simulink library "EdgePorts"  (R2022b)
settings: Solver=VariableStepAuto  StartTime=0.0  StopTime=10.0  RelTol=1e-3
libraries: HandyTextFile x5, AudioStats x4, $bdroot x2, TalariaApiBuffer x2
settings Model: Creator=kl13806  LastModifiedBy=kl13806
settings SolverCC: AlgebraicLoopSolver=TrustRegion
settings DebuggingCC: UnconnectedInputMsg=warning  UnconnectedOutputMsg=warning  UnconnectedLineMsg=warning  SFMachineParentedDataDiag=warning
settings ModelReferenceCC: EnableRefExpFcnMdlSchedulingChecks=on
settings RTWCC: DLArmComputeVersion=19.05

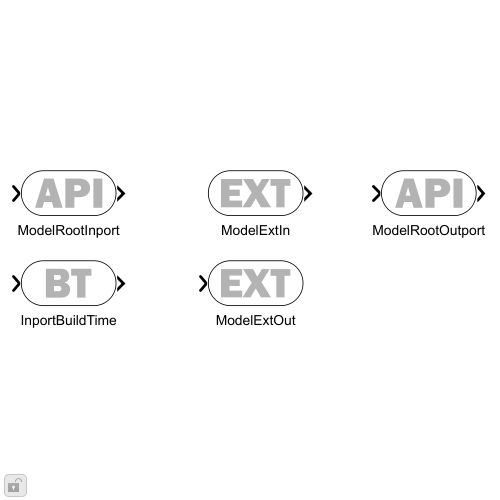
[thumbnail: Simulink's stored preview of the top-level diagram]
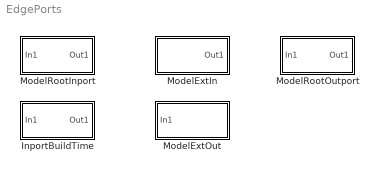
== system EdgePorts ==
  InportBuildTime : Subsystem  mask(Talaria Build-Time Configured Inport){Config=[]}
      mask prompts: Config "InportBuildTimeConfig"
      mask help: This block is just an inport with its signal attributes controlled by a build-time configuration object of type InportBTConfig.
      mask init:
      | blkh=gcbh;
      | Config=BTConfig.Assert(blkh,Config);
      | 
      | Config.Validate();
      mask Help: Supply the name of variable of type InportBTConfig in the mask dialog. Supplying empty (i.e. [ ]) will use class defaults which may change over time.
      mask Display: image('InportBT_Mask.svg'); % Use "Edit Image" on toolstrip to change.
  ModelExtIn : Subsystem  mask(Talaria Model External Inport){Config=[]}
      mask prompts: Config "ModelExtInConfig"
      mask help: This block acts like an inport and generates DLL API code.
      mask init:
      | blkh=gcbh;
      | Config=BTConfig.Assert(blkh,Config);
      | 
      | Config.Validate();
      mask Help:
      | The Talaria Model External Inport block assists with running algorithms which are built into DLLs. This block acts like an inport and exposes an API designed to feed data into the model. A driving program (e.g. a tuning tool) can use this standard interface to run any algorithm that uses this block.
      | 
      | See ext_port_model.m for an example of how to interface with the generated DLL. Also check the generated TalariaAPI.h source file.
      mask Display: image('ModelExtMask.svg'); % Use "Edit Image" on toolstrip to change.
  ModelExtOut : Subsystem  mask(Talaria Model External Outport){BufferName='Out1'}
      mask prompts: BufferName "Buffer Name:"
      mask help: This block acts like an outport and generates DLL API code.
      mask Help:
      | The Talaria Model External Outport block assists with running algorithms which are built into DLLs. This block acts like an outport and exposes an API designed to retrieve the data emit from the model. A driving program (e.g. a tuning tool) can use this standard interface to run any algorithm that uses this block.
      | 
      | See ext_port_model.m for an example of how to interface with the generated DLL. Also check the generated TalariaAPI.h source file.
      mask Display: image('ModelExtMask.svg'); % Use "Edit Image" on toolstrip to change.
  ModelRootInport : Subsystem  mask(Talaria Model Root Inport){Config=[]}
      mask prompts: Config "ModelRootInportConfig"
      mask help: This block controls the signal attributes, name, and storage class of attached buffer in the generated code. Also the buffer is surfaced as a model-level integration point (e.g. TalariaAPI.h, etc)
      mask init:
      | blkh=gcbh;
      | Config=BTConfig.Assert(blkh,Config);
      | 
      | Config.Validate();
      mask Help:
      | This block is intended to be used for root-block-diagram ports in an application model. Driven by built-time configuration, it sets up the input buffer's signal attributes, the type of buffer (e.g. extern pointer vs. exported model-allocated), and adds these specfications to the generated code in TalariaAPI.h.
      | 
      | Make sure to feed this block with just a normal Simulink root-level inport with no signal attributes settings made to it. All the configuration settings are asserted inside this block.
      mask Display: image('ModelRootInportMask.svg'); % Use "Edit Image" on toolstrip to change.
  ModelRootOutport : Subsystem  mask(Talaria Model Root Outport){Config=[]}
      mask prompts: Config "ModelRootOutportConfig"
      mask help: This block controls the name and storage class of attached buffer in the generated code. Also the buffer is surfaced as a model-level integration point (e.g. TalariaAPI.h, etc)
      mask init:
      | blkh=gcbh;
      | Config=BTConfig.Assert(blkh,Config);
      | 
      | Config.Validate();
      mask Help:
      | This block is intended to be used for root-block-diagram ports in an application model. Driven by built-time configuration, it sets up the output buffer qualities such as the type of buffer (e.g. extern pointer vs. exported model-allocated), and adds the discovered signal specfications to the generated code in TalariaAPI.h.
      | 
      | Note that this block does *not* control the signal attributes of the buffer such as data type, dimensions, and sample time.
      mask Display: image('ModelRootInportMask.svg'); % Use "Edit Image" on toolstrip to change.

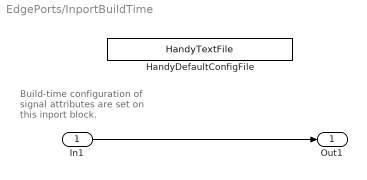
== system EdgePorts/InportBuildTime ==
  note: Build-time configuration of
      | signal attributes are set on
      | this inport block.
  In1 : Inport  OutDataTypeStr=Config.DataType  PortDimensions=Config.Dimensions  SampleTime=Config.SampleTime
  HandyDefaultConfigFile : HandyTextFile/HandyTextFile  TemplateSource=Config  FileSuffix=Config.m  OpenDialogOnLoad=off  UseThisBlockName=off  TheDefaultText=|  ShowInLibBrowser=on
      | classdef $(PREFIX)$(SUFFIX)
      | % $(FILENAME) Class definition to contain build-time configuration for $(PREFIX)
      | % Usage:
      | %    aConfig = $(PREFIX)$(SUFFIX)
      | %
      | 
      | %   Copyright 2020 Bose Corporation
      | 
      |   properties
      |     % Properties use this syntax:
      |     %    PropertyName size class {validation functions} = DefaultValue
      |     % About Build-Time Configuration: https://wiki.bose.com/x/dqPoB
      | 
      |     % Delete these examples:
      |     %Gain = 0.5
      |     %Theta = sin(pi/12)
      |     %MyDoubleArray (1,7) double {mustBeFinite} = [1 2 3 4 5 6 7]
      |     %LeftConfig (1,1) SubBlockConfig
      |     %RightConfig (1,1) SubBlockConfig
      | 
      |   end
      | end
      settings: SourceProductName=Bose Talaria
  Out1 : Outport
  wires:
  In1/1 -> Out1/1

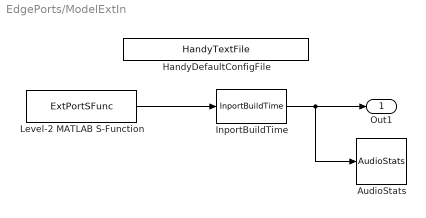
== system EdgePorts/ModelExtIn ==
  AudioStats : AudioStats/AudioStats  DoSampleRate=off  TypeSampleRate=Inherit: auto  DoCallRate=off  TypeCallRate=Inherit: auto  DoFrameSize=off  TypeFrameSize=Inherit: auto  DoChannelCount=off  TypeChannelCount=Inherit: auto  DoTaskRateFactor=off  TypeTaskRateFactor=Inherit: auto  MacroNameRoot=AUDIO  MacroNameRootEval=Config.BufferName  IsMacroNameEval=on  MacroSampleRate=on  MacroCallRate=on  MacroFrameSize=on  MacroChannelCount=on  MacroTaskRateFactor=on  MacroTaskId=on  ValidateSampleRate=off  ValueSampleRate=[]  ValidateCallRate=off  ValueCallRate=[]  ValidateFrameSize=off  ValueFrameSize=[]  ValidateChannelCount=off  ValueChannelCount=[]  ValidateTaskRateFactor=off  ValueTaskRateFactor=[]
      settings: SourceProductName=Bose Talaria
  HandyDefaultConfigFile : HandyTextFile/HandyTextFile  TemplateSource=Config  FileSuffix=Config.m  OpenDialogOnLoad=off  UseThisBlockName=off  TheDefaultText=|  ShowInLibBrowser=on
      | classdef $(PREFIX)$(SUFFIX)
      | % $(FILENAME) Class definition to contain build-time configuration for $(PREFIX)
      | % Usage:
      | %    aConfig = $(PREFIX)$(SUFFIX)
      | %
      | 
      | %   Copyright 2020 Bose Corporation
      | 
      |   properties
      |     % Properties use this syntax:
      |     %    PropertyName size class {validation functions} = DefaultValue
      |     % About Build-Time Configuration: https://wiki.bose.com/x/dqPoB
      | 
      |     % Delete these examples:
      |     %Gain = 0.5
      |     %Theta = sin(pi/12)
      |     %MyDoubleArray (1,7) double {mustBeFinite} = [1 2 3 4 5 6 7]
      |     %LeftConfig (1,1) SubBlockConfig
      |     %RightConfig (1,1) SubBlockConfig
      | 
      |   end
      | end
      settings: SourceProductName=Bose Talaria
  InportBuildTime : $bdroot/InportBuildTime  Config=Config
  Level-2 MATLAB S-Function : M-S-Function  FunctionName=ExtPortSFunc  Parameters=Config.BufferName,1
  Out1 : Outport
  wires:
  Level-2 MATLAB S-Function/1 -> InportBuildTime/1
  InportBuildTime/1 -> AudioStats/1, Out1/1

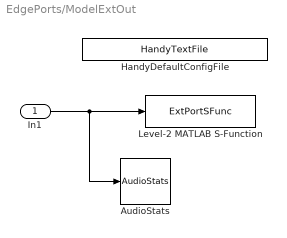
== system EdgePorts/ModelExtOut ==
  In1 : Inport
  AudioStats : AudioStats/AudioStats  DoSampleRate=off  TypeSampleRate=Inherit: auto  DoCallRate=off  TypeCallRate=Inherit: auto  DoFrameSize=off  TypeFrameSize=Inherit: auto  DoChannelCount=off  TypeChannelCount=Inherit: auto  DoTaskRateFactor=off  TypeTaskRateFactor=Inherit: auto  MacroNameRoot=AUDIO  MacroNameRootEval=BufferName  IsMacroNameEval=on  MacroSampleRate=on  MacroCallRate=on  MacroFrameSize=on  MacroChannelCount=on  MacroTaskRateFactor=on  MacroTaskId=on  ValidateSampleRate=off  ValueSampleRate=[]  ValidateCallRate=off  ValueCallRate=[]  ValidateFrameSize=off  ValueFrameSize=[]  ValidateChannelCount=off  ValueChannelCount=[]  ValidateTaskRateFactor=off  ValueTaskRateFactor=[]
      settings: SourceProductName=Bose Talaria
  HandyDefaultConfigFile : HandyTextFile/HandyTextFile  TemplateSource=Config  FileSuffix=Config.m  OpenDialogOnLoad=off  UseThisBlockName=off  TheDefaultText=|  ShowInLibBrowser=on
      | classdef $(PREFIX)$(SUFFIX)
      | % $(FILENAME) Class definition to contain build-time configuration for $(PREFIX)
      | % Usage:
      | %    aConfig = $(PREFIX)$(SUFFIX)
      | %
      | 
      | %   Copyright 2020 Bose Corporation
      | 
      |   properties
      |     % Properties use this syntax:
      |     %    PropertyName size class {validation functions} = DefaultValue
      |     % About Build-Time Configuration: https://wiki.bose.com/x/dqPoB
      | 
      |     % Delete these examples:
      |     %Gain = 0.5
      |     %Theta = sin(pi/12)
      |     %MyDoubleArray (1,7) double {mustBeFinite} = [1 2 3 4 5 6 7]
      |     %LeftConfig (1,1) SubBlockConfig
      |     %RightConfig (1,1) SubBlockConfig
      | 
      |   end
      | end
      settings: SourceProductName=Bose Talaria
  Level-2 MATLAB S-Function : M-S-Function  FunctionName=ExtPortSFunc  Parameters=BufferName,0
  wires:
  In1/1 -> AudioStats/1, Level-2 MATLAB S-Function/1

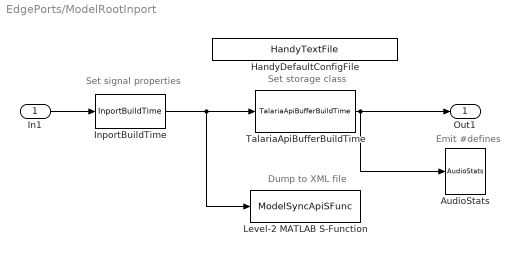
== system EdgePorts/ModelRootInport ==
  note: Dump to XML file
  note: Set storage class
  note: Set signal properties
  note: Emit #defines
  In1 : Inport
  AudioStats : AudioStats/AudioStats  DoSampleRate=off  TypeSampleRate=Inherit: auto  DoCallRate=off  TypeCallRate=Inherit: auto  DoFrameSize=off  TypeFrameSize=Inherit: auto  DoChannelCount=off  TypeChannelCount=Inherit: auto  DoTaskRateFactor=off  TypeTaskRateFactor=Inherit: auto  MacroNameRoot=AUDIO  MacroNameRootEval=Config.BufferName  IsMacroNameEval=on  MacroSampleRate=on  MacroCallRate=on  MacroFrameSize=on  MacroChannelCount=on  MacroTaskRateFactor=on  MacroTaskId=on  ValidateSampleRate=off  ValueSampleRate=[]  ValidateCallRate=off  ValueCallRate=[]  ValidateFrameSize=off  ValueFrameSize=[]  ValidateChannelCount=off  ValueChannelCount=[]  ValidateTaskRateFactor=off  ValueTaskRateFactor=[]
      settings: SourceProductName=Bose Talaria
  HandyDefaultConfigFile : HandyTextFile/HandyTextFile  TemplateSource=Config  FileSuffix=Config.m  OpenDialogOnLoad=off  UseThisBlockName=off  TheDefaultText=|  ShowInLibBrowser=on
      | classdef $(PREFIX)$(SUFFIX)
      | % $(FILENAME) Class definition to contain build-time configuration for $(PREFIX)
      | % Usage:
      | %    aConfig = $(PREFIX)$(SUFFIX)
      | %
      | 
      | %   Copyright 2020 Bose Corporation
      | 
      |   properties
      |     % Properties use this syntax:
      |     %    PropertyName size class {validation functions} = DefaultValue
      |     % About Build-Time Configuration: https://wiki.bose.com/x/dqPoB
      | 
      |     % Delete these examples:
      |     %Gain = 0.5
      |     %Theta = sin(pi/12)
      |     %MyDoubleArray (1,7) double {mustBeFinite} = [1 2 3 4 5 6 7]
      |     %LeftConfig (1,1) SubBlockConfig
      |     %RightConfig (1,1) SubBlockConfig
      | 
      |   end
      | end
      settings: SourceProductName=Bose Talaria
  InportBuildTime : $bdroot/InportBuildTime  Config=Config
  Level-2 MATLAB S-Function : M-S-Function  FunctionName=ModelSyncApiSFunc  Parameters=Config.BufferName,1,char(Config.AccessType)
  TalariaApiBufferBuildTime : TalariaApiBuffer/TalariaApiBufferBuildTime  Config=Config  TriggerInit=[415 69 515 111]
      settings: SourceProductName=Bose Talaria
  Out1 : Outport
  wires:
  In1/1 -> InportBuildTime/1
  InportBuildTime/1 -> Level-2 MATLAB S-Function/1, TalariaApiBufferBuildTime/1
  TalariaApiBufferBuildTime/1 -> AudioStats/1, Out1/1

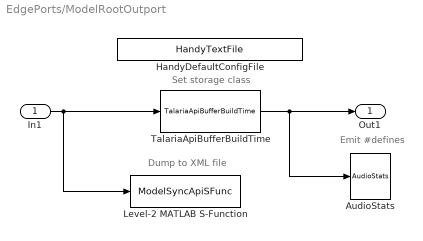
== system EdgePorts/ModelRootOutport ==
  note: Set storage class
  note: Dump to XML file
  note: Emit #defines
  In1 : Inport
  AudioStats : AudioStats/AudioStats  DoSampleRate=off  TypeSampleRate=Inherit: auto  DoCallRate=off  TypeCallRate=Inherit: auto  DoFrameSize=off  TypeFrameSize=Inherit: auto  DoChannelCount=off  TypeChannelCount=Inherit: auto  DoTaskRateFactor=off  TypeTaskRateFactor=Inherit: auto  MacroNameRoot=AUDIO  MacroNameRootEval=Config.BufferName  IsMacroNameEval=on  MacroSampleRate=on  MacroCallRate=on  MacroFrameSize=on  MacroChannelCount=on  MacroTaskRateFactor=on  MacroTaskId=on  ValidateSampleRate=off  ValueSampleRate=[]  ValidateCallRate=off  ValueCallRate=[]  ValidateFrameSize=off  ValueFrameSize=[]  ValidateChannelCount=off  ValueChannelCount=[]  ValidateTaskRateFactor=off  ValueTaskRateFactor=[]
      settings: SourceProductName=Bose Talaria
  HandyDefaultConfigFile : HandyTextFile/HandyTextFile  TemplateSource=Config  FileSuffix=Config.m  OpenDialogOnLoad=off  UseThisBlockName=off  TheDefaultText=|  ShowInLibBrowser=on
      | classdef $(PREFIX)$(SUFFIX)
      | % $(FILENAME) Class definition to contain build-time configuration for $(PREFIX)
      | % Usage:
      | %    aConfig = $(PREFIX)$(SUFFIX)
      | %
      | 
      | %   Copyright 2020 Bose Corporation
      | 
      |   properties
      |     % Properties use this syntax:
      |     %    PropertyName size class {validation functions} = DefaultValue
      |     % About Build-Time Configuration: https://wiki.bose.com/x/dqPoB
      | 
      |     % Delete these examples:
      |     %Gain = 0.5
      |     %Theta = sin(pi/12)
      |     %MyDoubleArray (1,7) double {mustBeFinite} = [1 2 3 4 5 6 7]
      |     %LeftConfig (1,1) SubBlockConfig
      |     %RightConfig (1,1) SubBlockConfig
      | 
      |   end
      | end
      settings: SourceProductName=Bose Talaria
  Level-2 MATLAB S-Function : M-S-Function  FunctionName=ModelSyncApiSFunc  Parameters=Config.BufferName,0,char(Config.AccessType)
  TalariaApiBufferBuildTime : TalariaApiBuffer/TalariaApiBufferBuildTime  Config=Config  TriggerInit=[415 69 515 111]
      settings: SourceProductName=Bose Talaria
  Out1 : Outport
  wires:
  TalariaApiBufferBuildTime/1 -> Out1/1, AudioStats/1
  In1/1 -> Level-2 MATLAB S-Function/1, TalariaApiBufferBuildTime/1
